simulink model "Modello_Dirigibile_Imbardata"  (R2013a)
settings: Solver=ode45  StartTime=0.0  StopTime=10.0  RelTol=1e-3
undefined symbols (not defined in the file): m
settings Model: Creator=Pera  LastModifiedBy=Pera

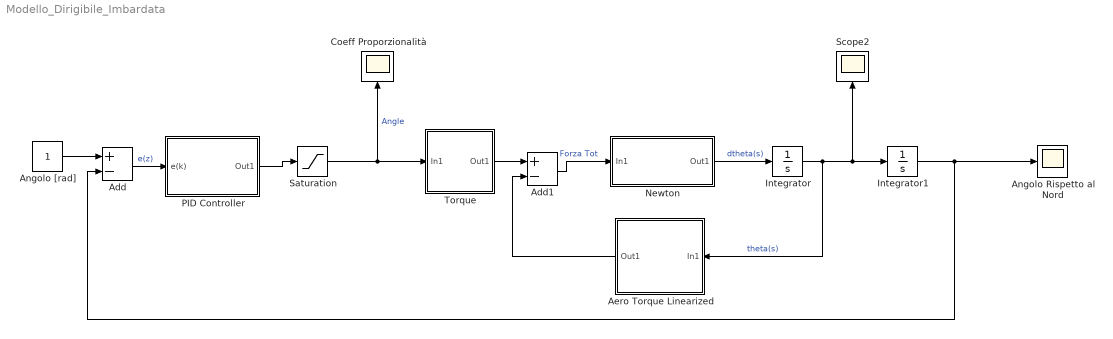
== system Modello_Dirigibile_Imbardata ==
  Add : Sum  Inputs=+-
  Add1 : Sum  Inputs=+-
  Aero Torque Linearized : Subsystem  mask{rho=1.225, radius=0.5, cd=0.5, d=0.5}
      mask prompts: rho "density"; cd "drag coeff"; d "baricentro-centro pallone"
      mask init:
      | s1=['rho= ',num2str(rho)];
      | s2=['radius= ',num2str(radius)];
      | s3=['cd= ',num2str(cd)];
      | s4=['d= ',num2str(d)];
      | s=strvcat(s1,s2,s3,s4);  %sto concatenando verticalmente
      mask Display: disp(s)
  Angolo Rispetto al Nord : Scope
  Angolo [rad] : Constant
  Coeff Proporzionalità : Scope
      settings: MaxDataPoints=10000
  Integrator : Integrator
  Integrator1 : Integrator
  Newton : Subsystem  mask{J=1}
      mask prompts: J "Inertia"
      mask init:
      | s=['Inertia= ',num2str(J),' [Kg*m^2]'];
      mask Display: disp(s)
  PID Controller : Subsystem  mask{Ts=0.2, kp=1.5, ki=0.2, kd=2}
      mask prompts: Ts "Sample Time"; kp "Guadagno Proporzionale"; ki "Guadagno Integrativo"; kd "Guadagno Derivativo"
      mask init:
      | s1=['kp= ',num2str(kp)];
      | s2=['ki= ',num2str(ki)];
      | s3=['kd= ',num2str(kd)];
      | s=strvcat(s1,s2,s3);  %sto concatenando verticalmente
      mask Display: disp(s)
  Saturation : Saturate  UpperLimit=2  LowerLimit=0
  Scope2 : Scope
      settings: SaveName=ScopeData2  MaxDataPoints=10000
  Torque : Subsystem  mask{T=0.6}
      mask prompts: T "Spinta"
      mask init:
      | s=['T= ',num2str(T),' [N]'];
      mask Display: disp(s)
  wires:
  Add/1 -> PID Controller/1(e(k))  "e(z)"
  Newton/1(Out1) -> Integrator/1  "dtheta(s)"
  Integrator/1 -> Aero Torque Linearized/1(In1), Integrator1/1, Scope2/1  "theta(s)"
  PID Controller/1(Out1) -> Saturation/1
  Saturation/1 -> Torque/1(In1), Coeff Proporzionalità/1  "Angle"
  Add1/1 -> Newton/1(In1)  "Forza Tot"
  Aero Torque Linearized/1(Out1) -> Add1/2
  Angolo [rad]/1 -> Add/1
  Torque/1(Out1) -> Add1/1
  Integrator1/1 -> Add/2, Angolo Rispetto al Nord/1

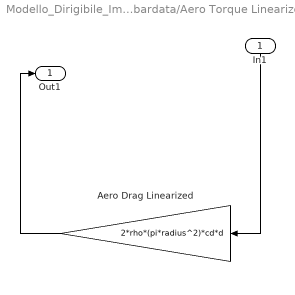
== system Modello_Dirigibile_Imbardata/Aero Torque Linearized ==
  In1 : Inport
  Aero Drag Linearized : Gain  Gain=2*rho*(pi*radius^2)*cd*d
  Out1 : Outport
  wires:
  In1/1 -> Aero Drag Linearized/1
  Aero Drag Linearized/1 -> Out1/1

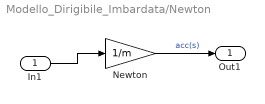
== system Modello_Dirigibile_Imbardata/Newton ==
  In1 : Inport
  Newton : Gain  Gain=1/m
  Out1 : Outport
  wires:
  In1/1 -> Newton/1
  Newton/1 -> Out1/1  "acc(s)"

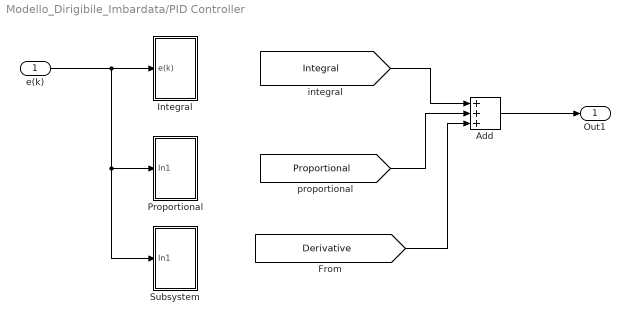
== system Modello_Dirigibile_Imbardata/PID Controller ==
  e(k) : Inport
  Add : Sum  Inputs=+++
  Integral : Subsystem
  Proportional : Subsystem
  Subsystem : Subsystem
  Out1 : Outport
  wires:
  [Integral] -> Add/1
  Add/1 -> Out1/1
  [Proportional] -> Add/2
  e(k)/1 -> Subsystem/1(In1), Proportional/1(In1), Integral/1(e(k))
  [Derivative] -> Add/3

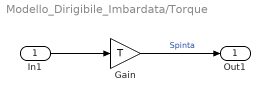
== system Modello_Dirigibile_Imbardata/Torque ==
  In1 : Inport
  Gain : Gain  Gain=T
  Out1 : Outport
  wires:
  Gain/1 -> Out1/1  "Spinta"
  In1/1 -> Gain/1

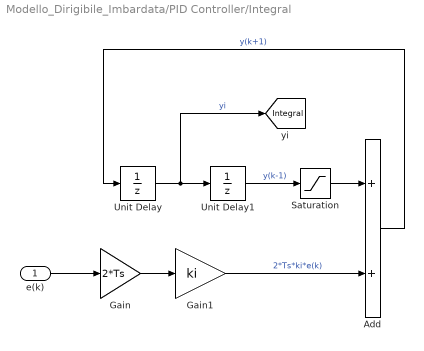
== system Modello_Dirigibile_Imbardata/PID Controller/Integral ==
  e(k) : Inport
  Add : Sum
  Gain : Gain  Gain=2*Ts
  Gain1 : Gain  Gain=ki
  Saturation : Saturate  UpperLimit=1  LowerLimit=-1
      settings: AttributesFormatString=|
      | %<LowerLimit>
      | %<UpperLimit>
  Unit Delay : UnitDelay  SampleTime=Ts
  Unit Delay1 : UnitDelay  SampleTime=Ts
  tag scope: Integral=global
  wires:
  Gain1/1 -> Add/2  "2*Ts*ki*e(k)"
  Unit Delay/1 -> [Integral], Unit Delay1/1  "yi"
  Gain/1 -> Gain1/1
  Saturation/1 -> Add/1
  Unit Delay1/1 -> Saturation/1  "y(k-1)"
  e(k)/1 -> Gain/1
  Add/1 -> Unit Delay/1  "y(k+1)"

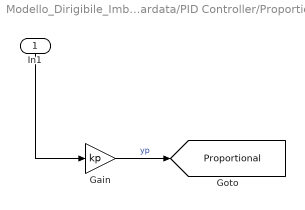
== system Modello_Dirigibile_Imbardata/PID Controller/Proportional ==
  In1 : Inport
  Gain : Gain  Gain=kp
  tag scope: Proportional=global
  wires:
  Gain/1 -> [Proportional]  "yp"
  In1/1 -> Gain/1

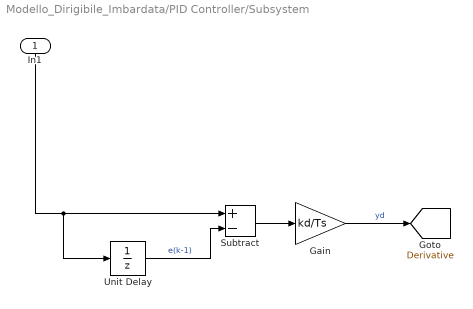
== system Modello_Dirigibile_Imbardata/PID Controller/Subsystem ==
  In1 : Inport
  Gain : Gain  Gain=kd/Ts
  Subtract : Sum  Inputs=+-
  Unit Delay : UnitDelay  SampleTime=-1
  tag scope: Derivative=global
  wires:
  Unit Delay/1 -> Subtract/2  "e(k-1)"
  Gain/1 -> [Derivative]  "yd"
  Subtract/1 -> Gain/1
  In1/1 -> Unit Delay/1, Subtract/1
